simulink library "Lib_Piccolo"  (R2018b)
settings: Solver=VariableStepAuto  StartTime=0.0  StopTime=10.0  RelTol=1e-3
values from neighbouring files (symbols this model uses):
  AccelErrInt2Brakes = 0.15    [SimulationControlConfig16P.m]    (also in SimulationControlConfig16P_F0.m; SimulationControlConfig16P_F2.m; SimulationControlConfig16P_LEGACY.m; SimulationControlConfigTAILLESS.m = 0.2)
  AileronMax = 25    [SimulationControlConfig16P.m]    (also in SimulationControlConfig16P_F0.m; SimulationControlConfig16P_F2.m; SimulationControlConfig16P_LEGACY.m; SimulationControlConfigTAILLESS.m)
  AileronPower = 0.00268    [SimulationControlConfig16P.m]    (also in SimulationControlConfig16P_F0.m; SimulationControlConfig16P_F2.m; SimulationControlConfig16P_LEGACY.m; SimulationControlConfigTAILLESS.m = 0.002266)
  AileronSurfaceMax = 45    [SimulationControlConfig16P.m]    (also in SimulationControlConfig16P_F0.m; SimulationControlConfig16P_F2.m; SimulationControlConfig16P_LEGACY.m; SimulationControlConfigTAILLESS_CGAFT_F0.m = 25)
  AileronTrim = 0    [SimulationControlConfig16P.m]    (also in SimulationControlConfig16P_F0.m; SimulationControlConfig16P_F2.m; SimulationControlConfig16P_LEGACY.m; SimulationControlConfigTAILLESS.m)
  Alt = 1000 + TerrainHeight    [SimulationStateConfig.m]
  AltCruise_m = Alt * 0.3048    [SimulationControlConfig16P.m]    (also in SimulationControlConfig16P_F2.m; SimulationControlConfigTAILLESS.m = Alt/3.28084; SimulationControlConfigTAILLESS_CGAFT_F0.m = 640; SimulationControlConfigTAILLESS_CGFWD_F0.m = 640)
  AltitudeRate2PitchCmdIntegratorInit = 0.1    [SimulationControlPre.m]
  AltMax = 10000    [SimulationControlConfig16P.m]    (also in SimulationControlConfig16P_F0.m; SimulationControlConfig16P_F2.m; SimulationControlConfig16P_LEGACY.m; SimulationControlConfigTAILLESS.m)
  AltMaxAccel = 2.5    [SimulationControlConfig16P.m]    (also in SimulationControlConfig16P_F0.m = 2; SimulationControlConfig16P_F2.m = 2; SimulationControlConfig16P_LEGACY.m = 0.9; SimulationControlConfigTAILLESS.m = 2)
  AltMin = 0    [SimulationControlConfig16P.m]    (also in SimulationControlConfig16P_F0.m; SimulationControlConfig16P_F2.m; SimulationControlConfig16P_LEGACY.m; SimulationControlConfigTAILLESS.m)
  AltRateCmd2Pitch = 0.26    [SimulationControlConfig16P.m]    (also in SimulationControlConfig16P_F0.m = 0.35; SimulationControlConfig16P_F2.m = 0.35; SimulationControlConfig16P_LEGACY.m = 0.6; SimulationControlConfigTAILLESS.m = 0.9)
  AltRateError2Pitch = 0.34    [SimulationControlConfig16P.m]    (also in SimulationControlConfig16P_F0.m = 0.61; SimulationControlConfig16P_F2.m = 0.61; SimulationControlConfig16P_LEGACY.m = 0.4; SimulationControlConfigTAILLESS.m = 0.3)
  AltRateErrorInt2Pitch = 0.61    [SimulationControlConfig16P.m]    (also in SimulationControlConfig16P_F0.m = 0.28; SimulationControlConfig16P_F2.m = 0.28; SimulationControlConfig16P_LEGACY.m = 0.45; SimulationControlConfigTAILLESS.m = 0.15)
  AltRateLpfCutOff = 3    [SimulationControlConfig16P.m]    (also in SimulationControlConfig16P_F0.m; SimulationControlConfig16P_F2.m; SimulationControlConfig16P_LEGACY.m; SimulationControlConfigTAILLESS.m = 5)
  AutoNosegear2Rudder = 26    [SimulationControlConfig16P.m]    (also in SimulationControlConfig16P_F0.m; SimulationControlConfig16P_F2.m; SimulationControlConfig16P_LEGACY.m; SimulationControlConfigTAILLESS.m = 25.2)
  b = 5.54    [SimulationControlConfig16P.m]    (also in SimulationControlConfig16P_F0.m; SimulationControlConfig16P_F2.m; SimulationControlConfig16P_LEGACY.m; SimulationControlConfigTAILLESS.m = 2.37)
  Bank2AileronIntegratorInit = 0    [SimulationControlPre.m]
  BankMax_User = BankMax_User/180*pi    (= 0.610865238198)    [SimulationControlConfig16P.m]    (also in SimulationControlConfig16P_F0.m = 0.523598775598; SimulationControlConfig16P_F2.m = 0.523598775598; SimulationControlConfig16P_LEGACY.m = 0.523598775598; SimulationControlConfigTAILLESS.m = 0.558505360638)
  baseLegFlaps = 20    [SimulationControlConfig16P.m]    (also in SimulationControlConfig16P_F0.m; SimulationControlConfig16P_F2.m = 15; SimulationControlConfig16P_LEGACY.m = 0; SimulationControlConfigTAILLESS.m = 0)
  C = GeneticOpt.C    [SimulationCostFunction.m]
  c = Sw/b    (= 0.841696750903)    [SimulationControlConfig16P.m]    (also in SimulationControlConfig16P_F0.m; SimulationControlConfig16P_F2.m; SimulationControlConfig16P_LEGACY.m; SimulationControlConfigTAILLESS.m = 0.354008438819)
  cell2WheelFactorMG = 5.98    [SimulationSensorConfig16P_LEGACY.m]
  cell2WheelFactorNG = 1    [SimulationSensorConfig16P_LEGACY.m]
  cellSatMaxMG = 15000    [SimulationSensorConfig16P.m]    (also in SimulationSensorConfig16P_LEGACY.m; SimulationSensorConfigTAILLESS7P.m; SimulationSensorConfigUTAIL7P.m)
  cellSatMaxNG = 1000    [SimulationSensorConfig16P.m]    (also in SimulationSensorConfig16P_LEGACY.m; SimulationSensorConfigTAILLESS7P.m; SimulationSensorConfigUTAIL7P.m)
  cellSatMinMG = -15000    [SimulationSensorConfig16P.m]    (also in SimulationSensorConfig16P_LEGACY.m; SimulationSensorConfigTAILLESS7P.m; SimulationSensorConfigUTAIL7P.m)
  cellSatMinNG = -1000    [SimulationSensorConfig16P.m]    (also in SimulationSensorConfig16P_LEGACY.m; SimulationSensorConfigTAILLESS7P.m; SimulationSensorConfigUTAIL7P.m)
  CL_Limit = CL_Max    (= 0.54)    [SimulationControlConfig16P.m]    (also in SimulationControlConfig16P_F0.m; SimulationControlConfig16P_F2.m = 0.638; SimulationControlConfig16P_LEGACY.m; SimulationControlConfigTAILLESS.m = 0.525)
  CL_Max = 0.54    [SimulationControlConfig16P.m]    (also in SimulationControlConfig16P_F0.m; SimulationControlConfig16P_F2.m = 0.638; SimulationControlConfig16P_LEGACY.m; SimulationControlConfigTAILLESS.m = 0.525)
  CL_Max_Nom = 0.465    [SimulationControlConfig16P.m]    (also in SimulationControlConfig16P_F0.m; SimulationControlConfig16P_F2.m = 0.563; SimulationControlConfig16P_LEGACY.m; SimulationControlConfigTAILLESS.m = 0.39)
  CL_Min = 0    [SimulationControlConfig16P.m]    (also in SimulationControlConfig16P_F0.m; SimulationControlConfig16P_F2.m; SimulationControlConfig16P_LEGACY.m; SimulationControlConfigTAILLESS.m)
  ClimbMaxFraction = 0.35    [SimulationControlConfig16P.m]    (also in SimulationControlConfig16P_F0.m = 0.17; SimulationControlConfig16P_F2.m = 0.17; SimulationControlConfig16P_LEGACY.m = 0.24; SimulationControlConfigTAILLESS.m = 0.21)
  ClimboutMaxBank = 7.0    (= 7)    [SimulationControlConfig16P.m]    (also in SimulationControlConfig16P_F0.m; SimulationControlConfig16P_F2.m; SimulationControlConfig16P_LEGACY.m; SimulationControlConfigTAILLESS.m = 5)
  ClimboutTimer = 7.0    (= 7)    [SimulationControlConfig16P.m]    (also in SimulationControlConfig16P_F0.m; SimulationControlConfig16P_F2.m; SimulationControlConfig16P_LEGACY.m; SimulationControlConfigTAILLESS.m)
  dCl_per_dFlap = 0.005581818    [SimulationControlConfig16P.m]    (also in SimulationControlConfig16P_F0.m = 0; SimulationControlConfig16P_F2.m = 0.0065; SimulationControlConfig16P_LEGACY.m = 0; SimulationControlConfigTAILLESS.m = 0)
  DecelerationCmd = 3.1    [SimulationControlConfig16P.m]    (also in SimulationControlConfig16P_F0.m; SimulationControlConfig16P_F2.m; SimulationControlConfig16P_LEGACY.m; SimulationControlConfigTAILLESS.m = 0.1)
  DeRotateLogicEndTimer = abs((NoseDownLimit_Deg-1)/DeRotateRamp_Dps)    [SimulationControlConfig16P.m]    (also in SimulationControlConfig16P_F0.m; SimulationControlConfig16P_F2.m; SimulationControlConfig16P_LEGACY.m; SimulationControlConfigTAILLESS.m)
  DeRotateLogicHoldNoseUpTimer = 0.1    [SimulationControlConfig16P.m]    (also in SimulationControlConfig16P_F0.m; SimulationControlConfig16P_F2.m; SimulationControlConfig16P_LEGACY.m; SimulationControlConfigTAILLESS.m)
  DeRotateLogicTimerTimeout = 2    [SimulationControlConfig16P.m]    (also in SimulationControlConfig16P_F0.m; SimulationControlConfig16P_F2.m; SimulationControlConfig16P_LEGACY.m; SimulationControlConfigTAILLESS.m)
  DeRotateLowerCmdSaturation = 0    [SimulationControlConfig16P.m]    (also in SimulationControlConfig16P_F0.m; SimulationControlConfig16P_F2.m; SimulationControlConfig16P_LEGACY.m; SimulationControlConfigTAILLESS.m)
  DeRotateRamp_Dps = 3    [SimulationControlConfig16P.m]    (also in SimulationControlConfig16P_F0.m; SimulationControlConfig16P_F2.m; SimulationControlConfig16P_LEGACY.m; SimulationControlConfigTAILLESS.m = 8)
  DeRotateUpperCmdSaturation = 7    [SimulationControlConfig16P.m]    (also in SimulationControlConfig16P_F0.m; SimulationControlConfig16P_F2.m; SimulationControlConfig16P_LEGACY.m; SimulationControlConfigTAILLESS.m)
  DescentMaxFraction = 0.22    [SimulationControlConfig16P.m]    (also in SimulationControlConfig16P_F0.m = 0.2; SimulationControlConfig16P_F2.m = 0.2; SimulationControlConfig16P_LEGACY.m = 0.2; SimulationControlConfigTAILLESS.m = 0.17)
  DesktopSimTerrainOffset_m = 0.406    [SimulationAircraftConfig.m]
  downwindFlaps = 0    [SimulationControlConfig16P.m]    (also in SimulationControlConfig16P_F0.m; SimulationControlConfig16P_F2.m = 15; SimulationControlConfig16P_LEGACY.m; SimulationControlConfigTAILLESS.m)
  downwindSplitAil = 0    [SimulationControlConfig16P_F2.m]
  DP_init = 0.5*1.225*V_init^2    [SimulationControlConfig16P.m]    (also in SimulationControlConfig16P_F0.m; SimulationControlConfig16P_F2.m; SimulationControlConfig16P_LEGACY.m; SimulationControlConfigTAILLESS.m)
  dscNoiseMG = 1    [SimulationSensorConfig16P_LEGACY.m]
  dscNoiseNG = 0.25    [SimulationSensorConfig16P_LEGACY.m]
  DSCnumBits = 24    [SimulationSensorConfig16P.m]    (also in SimulationSensorConfig16P_LEGACY.m; SimulationSensorConfigTAILLESS7P.m; SimulationSensorConfigUTAIL7P.m)
  DSCRangeMaxMG = 15000    [SimulationSensorConfig16P.m]    (also in SimulationSensorConfig16P_LEGACY.m; SimulationSensorConfigTAILLESS7P.m; SimulationSensorConfigUTAIL7P.m)
  DSCRangeMaxNG = 1000    [SimulationSensorConfig16P.m]    (also in SimulationSensorConfig16P_LEGACY.m; SimulationSensorConfigTAILLESS7P.m; SimulationSensorConfigUTAIL7P.m)
  DSCRangeMinMG = -15000    [SimulationSensorConfig16P.m]    (also in SimulationSensorConfig16P_LEGACY.m; SimulationSensorConfigTAILLESS7P.m; SimulationSensorConfigUTAIL7P.m)
  DSCRangeMinNG = -1000    [SimulationSensorConfig16P.m]    (also in SimulationSensorConfig16P_LEGACY.m; SimulationSensorConfigTAILLESS7P.m; SimulationSensorConfigUTAIL7P.m)
  dt = DLLSim.dt    [SimulationTimeStep.m]    (also in SimulationTrim.m = 0.02)
  EarlyTouchdownThreshold = 3.0    (= 3)    [SimulationControlConfig16P.m]    (also in SimulationControlConfig16P_F0.m; SimulationControlConfig16P_F2.m; SimulationControlConfig16P_LEGACY.m; SimulationControlConfigTAILLESS.m)
  ElevatorDeflectionRate = 15    [SimulationControlConfig16P.m]    (also in SimulationControlConfig16P_F0.m; SimulationControlConfig16P_F2.m; SimulationControlConfig16P_LEGACY.m = 12; SimulationControlConfigTAILLESS.m = 5)
  ElevatorMax = 25    [SimulationControlConfig16P.m]    (also in SimulationControlConfig16P_F0.m; SimulationControlConfig16P_F2.m; SimulationControlConfig16P_LEGACY.m; SimulationControlConfigTAILLESS.m)
  ElevatorPower = -0.002209    [SimulationControlConfig16P.m]    (also in SimulationControlConfig16P_F0.m; SimulationControlConfig16P_F2.m; SimulationControlConfig16P_LEGACY.m; SimulationControlConfigTAILLESS.m = -0.002668)
  ElevatorTrim = -3.5    [SimulationControlConfig16P.m]    (also in SimulationControlConfig16P_F0.m; SimulationControlConfig16P_F2.m; SimulationControlConfig16P_LEGACY.m; SimulationControlConfigTAILLESS.m = -3)
  elevonBias = 0    [SimulationControlConfig16P.m]    (also in SimulationControlConfig16P_F0.m; SimulationControlConfig16P_F2.m; SimulationControlConfig16P_LEGACY.m; SimulationControlConfigTAILLESS.m)
  Enable_TAS_Protection = 0    [SimulationControlConfig16P.m]    (also in SimulationControlConfig16P_F0.m; SimulationControlConfig16P_F2.m; SimulationControlConfig16P_LEGACY.m; SimulationControlConfigTAILLESS.m)
  EnableCrossTrackAbort = 1    [SimulationControlConfig16P.m]    (also in SimulationControlConfigTAILLESS.m; SimulationControlConfigTAILLESS_CGAFT_F0.m; SimulationControlConfigTAILLESS_CGFWD_F0.m; SimulationControlConfigTAILLESS_CGFWD_F2.m)
  EnergyBandwidth = 0.04    [SimulationControlConfig16P.m]    (also in SimulationControlConfig16P_F0.m = 0.03; SimulationControlConfig16P_F2.m = 0.03; SimulationControlConfig16P_LEGACY.m = 0.02; SimulationControlConfigTAILLESS.m = 0.06)
  EngineLhFuelCut = 0    [SimulationAircraftConfig.m]
  EngineRhFuelCut = 0    [SimulationAircraftConfig.m]
  FastThrottleRate = 0.075    [SimulationControlConfig16P.m]    (also in SimulationControlConfig16P_F0.m = 0.05; SimulationControlConfig16P_F2.m = 0.05; SimulationControlConfig16P_LEGACY.m = 0.05; SimulationControlConfigTAILLESS.m = 0.1)
  FilterWarmUpTime = 2    [SimulationSensorConfig16P.m]    (also in SimulationSensorConfig16P_LEGACY.m; SimulationSensorConfigTAILLESS7P.m; SimulationSensorConfigUTAIL7P.m)
  finalApproachFlaps = 20    [SimulationControlConfig16P.m]    (also in SimulationControlConfig16P_F0.m; SimulationControlConfig16P_F2.m = 15; SimulationControlConfig16P_LEGACY.m = 0; SimulationControlConfigTAILLESS.m = 0)
  finalApproachSplitAil = 20    [SimulationControlConfig16P_F2.m]
  FinalDescentSlope_Deg = testPlans(testIndx).descentSlope    [SimulationControlConfig16P.m]    (also in SimulationControlConfig16P_F0.m; SimulationControlConfig16P_F2.m; SimulationControlConfig16P_LEGACY.m; SimulationControlConfigTAILLESS.m)
  flapMax = 0    [SimulationControlConfig16P.m]    (also in SimulationControlConfig16P_F0.m = 35; SimulationControlConfig16P_F2.m = 33; SimulationControlConfig16P_LEGACY.m; SimulationControlConfigTAILLESS.m)
  flapRate = 7.5    [SimulationControlConfig16P.m]    (also in SimulationControlConfig16P_F0.m; SimulationControlConfig16P_F2.m; SimulationControlConfig16P_LEGACY.m; SimulationControlConfigTAILLESS.m = 6.6)
  FlareHeight = 5    [SimulationControlConfig16P.m]    (also in SimulationControlConfig16P_F0.m; SimulationControlConfig16P_F2.m; SimulationControlConfig16P_LEGACY.m = 4.8; SimulationControlConfigTAILLESS.m = 2.75)
  FlareVerticalRate_mps = -0.4    [SimulationControlConfig16P.m]    (also in SimulationControlConfig16P_F0.m; SimulationControlConfig16P_F2.m; SimulationControlConfig16P_LEGACY.m = -0.5; SimulationControlConfigTAILLESS.m = -0.15)
  Fp_Aileron = 0.55*2*pi*RollRateLpfCutoff*dt    [SimulationControlConfig16P.m]    (also in SimulationControlConfig16P_F0.m; SimulationControlConfig16P_F2.m; SimulationControlConfig16P_LEGACY.m; SimulationControlConfigTAILLESS.m)
  Fp_Alt = 2*pi*0.55*AltBandwidth    (= 0.622035345411)    [SimulationControlConfig16P.m]    (also in SimulationControlConfig16P_F0.m; SimulationControlConfig16P_F2.m; SimulationControlConfig16P_LEGACY.m = 0.099; SimulationControlConfigTAILLESS.m = 0.207345115137)
  Fp_AltRate = 0.55*2*pi*AltRateLpfCutOff*dt    [SimulationControlConfig16P.m]    (also in SimulationControlConfig16P_F0.m; SimulationControlConfig16P_F2.m; SimulationControlConfig16P_LEGACY.m; SimulationControlConfigTAILLESS.m)
  Fp_Elevator = 0.55*2*pi*PitchRateLpfCutoff*dt    [SimulationControlConfig16P.m]    (also in SimulationControlConfig16P_F0.m; SimulationControlConfig16P_F2.m; SimulationControlConfig16P_LEGACY.m; SimulationControlConfigTAILLESS.m)
  Fp_Energy = 0.55*2*pi*EnergyBandwidth    (= 0.138230076758)    [SimulationControlConfig16P.m]    (also in SimulationControlConfig16P_F0.m = 0.103672557568; SimulationControlConfig16P_F2.m = 0.103672557568; SimulationControlConfig16P_LEGACY.m = 0.069115038379; SimulationControlConfigTAILLESS.m = 0.207345115137)
  Fp_Energy2 = 0.55*2*pi*EnergyBandwidth*dt    [SimulationControlConfig16P.m]    (also in SimulationControlConfig16P_F0.m; SimulationControlConfig16P_F2.m; SimulationControlConfig16P_LEGACY.m; SimulationControlConfigTAILLESS.m)
  Fp_Pitch = 0.55*2*pi*PitchBandwidth    (= 2.45358386245)    [SimulationControlConfig16P.m]    (also in SimulationControlConfig16P_F0.m; SimulationControlConfig16P_F2.m = 1.72787595947; SimulationControlConfig16P_LEGACY.m = 3.11017672705; SimulationControlConfigTAILLESS.m = 1.55508836353)
  Fp_Pitch_2 = 0.55*2*pi*PitchBandwidth*dt    [SimulationControlConfig16P.m]    (also in SimulationControlConfig16P_F0.m; SimulationControlConfig16P_F2.m; SimulationControlConfig16P_LEGACY.m; SimulationControlConfigTAILLESS.m)
  Fp_Roll = RollBandwidth^2    (= 1.69)    [SimulationControlConfig16P.m]    (also in SimulationControlConfig16P_F0.m = 1.44; SimulationControlConfig16P_F2.m = 1.44; SimulationControlConfig16P_LEGACY.m = 1.44; SimulationControlConfigTAILLESS.m = 1.21)
  Fp_Rudder = 0.55*2*pi*YawRateLpfCutoff*dt    [SimulationControlConfig16P.m]    (also in SimulationControlConfig16P_F0.m; SimulationControlConfig16P_F2.m; SimulationControlConfig16P_LEGACY.m; SimulationControlConfigTAILLESS.m)
  Fp_TAS = 0.55*2*pi*TASBandwidth    (= 0.103672557568)    [SimulationControlConfig16P.m]    (also in SimulationControlConfig16P_F0.m; SimulationControlConfig16P_F2.m; SimulationControlConfig16P_LEGACY.m; SimulationControlConfigTAILLESS.m = 0.172787595947)
  Fp_TAS_Filter = 2*pi*TasLpfCutoff*dt    [SimulationControlConfig16P.m]    (also in SimulationControlConfig16P_F0.m; SimulationControlConfig16P_F2.m; SimulationControlConfig16P_LEGACY.m; SimulationControlConfigTAILLESS.m)
  Fp_Turn = 0.55*2*pi*TurnErrLPFcutoff    (= 0.172787595947)    [SimulationControlConfig16P.m]    (also in SimulationControlConfig16P_F0.m = 0.0345575191895; SimulationControlConfig16P_F2.m = 0.0345575191895; SimulationControlConfig16P_LEGACY.m = 0.0345575191895; SimulationControlConfigTAILLESS.m)
  Fp_TurnDerr = 0.55*2*pi*TurnDerivativeLPFcutoff    (= 0.172787595947)    [SimulationControlConfig16P.m]    (also in SimulationControlConfig16P_F0.m = 0.0345575191895; SimulationControlConfig16P_F2.m = 0.0345575191895; SimulationControlConfig16P_LEGACY.m = 0.0345575191895; SimulationControlConfigTAILLESS.m)
  FTV = 3    [SimulationAircraftConfig.m]
  ftvStaticPositionError = 1/1.18    (= 0.847457627119)    [SimulationSensorConfig16P.m]    (also in SimulationSensorConfig16P_LEGACY.m; SimulationSensorConfigTAILLESS7P.m = 1; SimulationSensorConfigUTAIL7P.m = 1)
  g = 9.81    [SimulationStateConfig.m]
  goAroundSplitAil = 0    [SimulationControlConfig16P_F2.m]
  GustSpd_Kts = testPlans(testIndx).gustSpd    [SimulationStateConfig.m]
  GustTriggerVal = testPlans(testIndx).gustTriggerVal    [SimulationStateConfig.m]
  HeadingErr2TurnRate = 0.5    [SimulationControlConfig16P.m]    (also in SimulationControlConfig16P_F0.m; SimulationControlConfig16P_F2.m; SimulationControlConfig16P_LEGACY.m; SimulationControlConfigTAILLESS.m)
  HeadingErrDer2TurnRate = 0.3    [SimulationControlConfig16P.m]    (also in SimulationControlConfig16P_F0.m; SimulationControlConfig16P_F2.m; SimulationControlConfig16P_LEGACY.m; SimulationControlConfigTAILLESS.m)
  IASbounce = IASstall*0.8    [SimulationControlPre.m]
  IAScruiseCMD = sqrt(2*m*9.81/(1.225*Sw*CL_cruise))    [SimulationControlConfig16P.m]    (also in SimulationControlConfig16P_F0.m; SimulationControlConfig16P_F2.m; SimulationControlConfig16P_LEGACY.m; SimulationControlConfigTAILLESS.m)
  IASfinalCMD = 1.12 * IASmin    [SimulationControlConfig16P.m]    (also in SimulationControlConfig16P_F0.m = 1.14 * IASmin; SimulationControlConfig16P_F2.m = 1.10 * IASmin; SimulationControlConfig16P_LEGACY.m = 1.10 * IASmin; SimulationControlConfigTAILLESS.m = 1.14 * IASmin)
  IASflareCMD = IASstall    [SimulationControlConfig16P.m]    (also in SimulationControlConfig16P_F0.m; SimulationControlConfig16P_F2.m; SimulationControlConfig16P_LEGACY.m; SimulationControlConfigTAILLESS.m)
  IASmax = 64    [SimulationControlConfig16P.m]    (also in SimulationControlConfig16P_F0.m = 46; SimulationControlConfig16P_F2.m = 52; SimulationControlConfig16P_LEGACY.m = 46; SimulationControlConfigTAILLESS.m = 38.9)
  IASmin = sqrt(2*m*9.81/(1.225*Sw*0.9*CL_Max_Nom))    [SimulationControlConfig16P.m]    (also in SimulationControlConfig16P_F0.m; SimulationControlConfig16P_F2.m; SimulationControlConfig16P_LEGACY.m; SimulationControlConfigTAILLESS.m)
  IASshortCMD = IASstall    [SimulationControlConfig16P.m]    (also in SimulationControlConfig16P_F0.m; SimulationControlConfig16P_F2.m; SimulationControlConfig16P_LEGACY.m; SimulationControlConfigTAILLESS.m)
  IASstall = sqrt(2*m*9.81/(1.225*Sw*CL_Max))    [SimulationControlConfig16P.m]    (also in SimulationControlConfig16P_F0.m; SimulationControlConfig16P_F2.m; SimulationControlConfig16P_LEGACY.m; SimulationControlConfigTAILLESS.m)
  inFlight = 1    [SimulationControlConfig16P.m]    (also in SimulationControlConfigTAILLESS.m; SimulationControlConfigTAILLESS_CGAFT_F0.m; SimulationControlConfigTAILLESS_CGFWD_F0.m; SimulationControlConfigTAILLESS_CGFWD_F2.m)
  JetCatOffset = 5    [SimulationControlConfig16P.m]    (also in SimulationControlConfig16P_F0.m; SimulationControlConfig16P_F2.m; SimulationControlConfig16P_LEGACY.m)
  LaunchRollingElevator = -1.5    [SimulationControlConfig16P.m]    (also in SimulationControlConfig16P_F0.m; SimulationControlConfig16P_F2.m = 1.25; SimulationControlConfig16P_LEGACY.m; SimulationControlConfigTAILLESS.m = 1)
  ldg_NosegearMax = 10    [SimulationControlConfig16P.m]    (also in SimulationControlConfig16P_F0.m; SimulationControlConfig16P_F2.m; SimulationControlConfig16P_LEGACY.m; SimulationControlConfigTAILLESS.m)
  ldg_TrackVyErrInt2Nosegear = 0.1250    (= 0.125)    [SimulationControlConfig16P.m]    (also in SimulationControlConfig16P_F0.m; SimulationControlConfig16P_F2.m; SimulationControlConfig16P_LEGACY.m; SimulationControlConfigTAILLESS.m = 0.00714285714286)
  ldg_TrackVyErrPro2Nosegear = 0.35    [SimulationControlConfig16P.m]    (also in SimulationControlConfig16P_F0.m; SimulationControlConfig16P_F2.m; SimulationControlConfig16P_LEGACY.m; SimulationControlConfigTAILLESS.m = 0.0546666666667)
  ldg_TrackY2Vy = 0.07    [SimulationControlConfig16P.m]    (also in SimulationControlConfig16P_F0.m; SimulationControlConfig16P_F2.m; SimulationControlConfig16P_LEGACY.m; SimulationControlConfigTAILLESS.m = 0.17)
  ldg_Vy2NosegearScalingPower = 1.075    [SimulationControlConfig16P.m]    (also in SimulationControlConfig16P_F0.m; SimulationControlConfig16P_F2.m; SimulationControlConfig16P_LEGACY.m; SimulationControlConfigTAILLESS.m = 0.6)
  ldg_Y2VyScalingPower = 0.175    [SimulationControlConfig16P.m]    (also in SimulationControlConfig16P_F0.m; SimulationControlConfig16P_F2.m; SimulationControlConfig16P_LEGACY.m; SimulationControlConfigTAILLESS.m = 0)
  ldg_YawRate2Nosegear = 0.175    [SimulationControlConfig16P.m]    (also in SimulationControlConfig16P_F0.m; SimulationControlConfig16P_F2.m; SimulationControlConfig16P_LEGACY.m; SimulationControlConfigTAILLESS.m = 0.065)
  LiftSlope = 0.064285    [SimulationControlConfig16P.m]    (also in SimulationControlConfig16P_F0.m; SimulationControlConfig16P_F2.m; SimulationControlConfig16P_LEGACY.m; SimulationControlConfigTAILLESS.m = 0.058631)
  LPFaileronInit = 0    [SimulationControlPre.m]
  LPFclestInit = 0    [SimulationControlPre.m]
  LPFenergyFFInit = 0    [SimulationControlPre.m]
  ... (+122 more)
undefined symbols (not defined in the file or in its folder): abortFlag, alphaHPF, apmDelay, BRWNOUT, CRAWOR, CRAWUR, DiscIntNeverNeededParam, DLLSim, DLLSimStep, ECOMOR, ECOMUR, Fp_Tas, GustTrigger_HeightAgl_m, IPSTAT, LCINTEG, Ldg_Persist_Time, LOWER_FLAGS, MSG_ENABLE, NoiseStd, OLDVAL, OVERRIDE_ENABLE, OVERRIDE_VALUE, REBOOT, reversionEnable, revIASMax, revIASMin, revPitchMax, revPitchMin, revPitchRateMax, revRollMax, revRollRateMax, SAMPLE, SCALON, SensorModel, sigbuilder_block, Sim_Vx, Sim_Vy, Sim_Vz, Sim_Xpos, Sim_Ypos, Sim_Zpos, SYSOR, SYSUR, TARE, TEMPOR, TEMPUR, testIndx, testPlan, testPlans, Trim_piccoloInCmd, Trim_REFSI_FD_IN_nmodeCgShifterCmd_Flag, Trim_REFSI_FD_IN_nmodeCgShifterCmd_Ft, Trim_REFSI_FD_IN_nmodeCgShifterCmdType, Trim_REFSI_FD_IN_nmodeCgShifterNRCActive, Trim_REFSI_FD_IN_nmodeFlapLhIBCmd_Deg, Trim_REFSI_FD_IN_nmodeFlapLhOBCmd_Deg, Trim_REFSI_FD_IN_nmodeFlapRhIBCmd_Deg, Trim_REFSI_FD_IN_nmodeFlapRhOBCmd_Deg, Trim_REFSI_FD_IN_nmodeSlatLhCmd_Deg ... (+11)
libraries: simulink x1237, $bdroot x179, aerolibconvert2 x63, dspswit3 x25, aerolibatmos2 x5, simulink_extras x4, dsparch4 x2, Lib_Piccolo_Alt x2, eeGeneralControl x1, dspindex x1
(part 24 of 74)

== system Lib_Piccolo/Emulated INS/Accelerometer Noise Model/Generate Accel Noise ==
  ContactBool : Inport
  gndSpeed_mps : Inport  Port=2
  Constant1 : Constant
  Constant2 : Constant  Value=10
  Data Type Conversion : DataTypeConversion
  Divide : Product  Inputs=*/
  Low-Pass Filter (Discrete or Continuous) : eeGeneralControl/Low-Pass Filter (Discrete or Continuous)  Commented=through  K=1  T=0.2  B=inf  A=-inf  init_option=Inherited from block input  x0=0  Ts=-1
  Multiply{,1..8} (9 alike) : Product
  Saturation3 : Saturate  UpperLimit=SensorModel.IMU.noiseScalarMax  LowerLimit=SensorModel.IMU.noiseScalarMin
  Sum : Sum  Inputs=+-|
  Sum1 : Sum
  Sum2 : Sum
  Sum3 : Sum
  xAccelNoiseInAir : RandomNumber  Variance=SensorModel.IMU.xAccelNoiseVarianceInAir
  xAccelNoiseOnGnd : RandomNumber  Variance=SensorModel.IMU.xAccelNoiseVarianceOnGnd
  yAccelNoiseInAir : RandomNumber  Variance=SensorModel.IMU.yAccelNoiseVarianceInAir
  yAccelNoiseOnGnd : RandomNumber  Variance=SensorModel.IMU.yAccelNoiseVarianceOnGnd
  zAccelNoiseInAir : RandomNumber  Variance=SensorModel.IMU.zAccelNoiseVarianceInAir
  zAccelNoiseOnGnd : RandomNumber  Variance=SensorModel.IMU.zAccelNoiseVarianceOnGnd
  NoiseXaccelmps2 : Outport
  NoiseYaccelmps2 : Outport  Port=2
  NoiseZaccelmps2 : Outport  Port=3
  wires:
  Sum1/1 -> Multiply8/1
  Multiply8/1 -> NoiseXaccelmps2/1
  Multiply7/1 -> NoiseYaccelmps2/1
  Sum2/1 -> Multiply7/1
  Multiply6/1 -> NoiseZaccelmps2/1
  Sum3/1 -> Multiply6/1
  Saturation3/1 -> Multiply6/2, Multiply7/2, Multiply8/2  "gndSpdScalar"
  Constant2/1 -> Divide/2
  Divide/1 -> Saturation3/1
  gndSpeed_mps/1 -> Divide/1
  ContactBool/1 -> Data Type Conversion/1
  Data Type Conversion/1 -> Low-Pass Filter (Discrete or Continuous)/1
  zAccelNoiseInAir/1 -> Multiply4/1
  Multiply5/1 -> Sum3/2
  Multiply4/1 -> Sum3/1
  zAccelNoiseOnGnd/1 -> Multiply5/2
  Multiply2/1 -> Sum2/1
  yAccelNoiseOnGnd/1 -> Multiply3/2
  yAccelNoiseInAir/1 -> Multiply2/1
  Multiply3/1 -> Sum2/2
  xAccelNoiseOnGnd/1 -> Multiply1/2
  xAccelNoiseInAir/1 -> Multiply/1
  Multiply1/1 -> Sum1/2
  Constant1/1 -> Sum/1
  Low-Pass Filter (Discrete or Continuous)/1 -> Sum/2, Multiply1/1, Multiply3/1, Multiply5/1  "onGnd"
  Sum/1 -> Multiply2/2, Multiply4/2, Multiply/2  "inAir"
  Multiply/1 -> Sum1/1

== system Lib_Piccolo/Ground Detection Systems/CL Detection Wrapper/CL Based Touchdown Detection Logic ==
  note: This is a latch used only in the touchdown, and rollout Piccolo Controller Modes
  note: When this is true Piccolo is indicating the WOW system armed.
  note: This is a latch used only in the short final, touchdown, and rollout Piccolo Controller Modes
  Pic_WOW : Inport
  Pic_APMode : Inport  Port=2
  CL : Inport  Port=3
  Compare To Constant1 : simulink/Logic and Bit Operations/Compare To Constant  relop=>  const=-1  OutDataTypeStr=uint8
  Compare To Constant2 : simulink/Logic and Bit Operations/Compare To Constant  relop=>=  const=10  OutDataTypeStr=uint8
  Compare To Constant6 : simulink/Logic and Bit Operations/Compare To Constant  relop=>=  const=9  OutDataTypeStr=uint8
  Constant : Constant  Value=EarlyTouchdownThreshold
  Constant1 : Constant  Value=TouchdownThreshold
  Constant10 : Constant  Value=0
  Constant2 : Constant  Value=CL_Max
  Constant3 : Constant  Value=0
  Constant4 : Constant
  Constant5 : Constant
  Constant6 : Constant  Value=0
  Constant7 : Constant  Value=TouchdownThreshold
  Constant8 : Constant  Value=2
  Constant9 : Constant
  Latch : Subsystem
  Latch1 : Subsystem
  Multiply{,1..4} (5 alike) : Product
  NOT : Logic  Operator=NOT  IconShape=distinctive  AllPortsSameDT=off  OutDataTypeStr=boolean
  Subtract : Sum  Inputs=-+
  Subtract1 : Sum  Inputs=-+
  Subtract2 : Sum  Inputs=+-
  Switch : Switch
  Switch1 : Switch
  Switch2 : Switch  Threshold=2
  Switch3 : Switch
  Switch4 : Switch  Criteria=u2 > Threshold
  EarlyTouchdownFlag : Outport
  TouchdownFlag : Outport  Port=2
  wires:
  Pic_WOW/1 -> Compare To Constant1/1
  Compare To Constant1/1 -> NOT/1
  Switch/1 -> Switch4/1
  Switch3/1 -> Switch4/3
  Constant5/1 -> Switch1/1
  Constant6/1 -> Switch1/3
  Constant4/1 -> Switch/1
  Multiply/1 -> Subtract1/1
  Constant1/1 -> Multiply1/2
  Constant/1 -> Multiply/2
  Constant3/1 -> Switch/3
  Subtract/1 -> Switch/2
  Subtract1/1 -> Switch1/2
  CL/1 -> Subtract2/1, Subtract1/2, Subtract/2
  Constant2/1 -> Multiply/1, Multiply2/1, Multiply1/1
  Multiply1/1 -> Subtract/1
  Constant7/1 -> Switch2/1, Switch2/2
  Switch2/1 -> Multiply2/2
  Multiply2/1 -> Subtract2/2
  Subtract2/1 -> Switch3/2
  Constant9/1 -> Switch3/1
  Constant10/1 -> Switch3/3
  Pic_APMode/1 -> Compare To Constant2/1, Compare To Constant6/1
  Switch1/1 -> Multiply3/1
  Constant8/1 -> Switch2/3
  NOT/1 -> Switch4/2
  Latch/1(Q_Latched) -> EarlyTouchdownFlag/1
  Latch1/1(Q_Latched) -> TouchdownFlag/1
  Compare To Constant2/1 -> Latch1/2(Enable/!Rst), Multiply4/2
  Compare To Constant6/1 -> Latch/2(Enable/!Rst), Multiply3/2
  Multiply3/1 -> Latch/1(D)
  Multiply4/1 -> Latch1/1(D)
  Switch4/1 -> Multiply4/1

== system Lib_Piccolo/Ground Detection Systems/WoW Wrapper/Variant Subsystem ==
  note: 16 - Logic derived from LOAD2, with key changes:
      | - Saturation on inputs to filter to prevent 'wind-up'
      | - Fix to signal probe location used to drive one-wheel and persistence chain (this is a change from LOAD14)
      |
      | NOTE - this variant of the model has updates & simplifications to model elements upstream of the K2 and correct representation of DSC resolution. Not propagated to previous variants!
  note: 1) Add Subsystem or Model blocks as valid variant choices.
      | 2) You cannot connect blocks at this level. At simulation, connectivity is automatically
      | determined, based on the active variant and port name matching.
  note: 18 - Core logic & modelling is matched to 16 , with updates to accomodate landing with single-wheel DSC failures.
  note: 20 - Detection logic is that of 16 with addition of single-wheel failure handling . System further developed in Simulink for test & code-generation capability.
  Piccolo_AP_Mode : Inport
  WoW_Bus_In : Inport  Port=2
  Load Cell WoW Model 1 : Subsystem  VariantControl="SensorModel.WOW.Cell.Variant==\"LOAD1\""  mask{Ldg_Persist_Time=SensorModel.WOW.Cell.persistanceTime_s, Ldg_Latch_Time_P=SensorModel.WOW.Cell.longLatchTime_s, Ldg_Latch_Time_S=SensorModel.WOW.Cell.shortLatchTime_s, Ldg_Load_Thresh_Upper=SensorModel.WOW.Cell.loadThresholdUpper_N, Ldg_Load_Thresh_Lower=SensorModel.WOW.Cell.loadThresholdLower_N, TO_Persist_Time=SensorModel.WOW.Cell.TO_persistanceTime_s, TO_Latch_Time=SensorModel.WOW.Cell.TO_latchTime_s, TO_Load_Thresh=SensorModel.WOW.Cell.TO_loadThreshold_N, DSCnumBits=24, numBits=16, satMaxMG=15000, satMinMG=-300, dscNoiseMG=1, DSCRangeMaxMG=15000, DSCRangeMinMG=-15000, satMaxNG=1000, satMinNG=-250, dscNoiseNG=0.25, DSCRangeMaxNG=1000, DSCRangeMinNG=-1000, cellSatMaxMG=15000, cellSatMinMG=-15000, cell2WheelFactorMG=5.98, cellSatMaxNG=1000, cellSatMinNG=-1000, cell2WheelFactorNG=1}
      mask prompts: Ldg_Persist_Time "Landing Persistance Time [s]"; Ldg_Latch_Time_P "Primary Landing Latch Time [s]"; Ldg_Latch_Time_S "Secondary Landing Latch Time [s]"; Ldg_Load_Thresh_Upper "Landing Load Threshold Upper [N]"; Ldg_Load_Thresh_Lower "Landing Load Threshold Lower [N]"; TO_Persist_Time "Take Off Persistance Time [s]"; TO_Latch_Time "Take Off Latch Time [s]"; TO_Load_Thresh "Take Off Load Threshold  [N]"; DSCnumBits "DSC Encoded Resolution [num bits]"; numBits "CANBridge Encoded Resolution [num bits]"; satMaxMG "Main Gear CANBridge Saturation Max [N]"; satMinMG "Main Gear CANBridge Saturation Min [N]"; dscNoiseMG "Main Gear DSC Noise Level pk-pk [N]"; DSCRangeMaxMG "Main Gear DSC Range Max [N]"; DSCRangeMinMG "Main Gear DSC Range Min [N]"; satMaxNG "Nose Gear CANBridge Saturation Max [N]"; satMinNG "Nose Gear CANBridge Saturation Min [N]"; dscNoiseNG "Nose Gear DSC Noise Level pk-pk [N]"; DSCRangeMaxNG "Nose Gear DSC Range Max [N]"; DSCRangeMinNG "Nose Gear DSC Range Min [N]"; cellSatMaxMG "Main Gear Cell Saturation Max [N]"; cellSatMinMG "Main Gear Cell Saturation Min [N]"; cell2WheelFactorMG "Main Gear Cell to Wheel Load Scale Factor"; cellSatMaxNG "Nose Gear Cell Saturation Max [N]"; cellSatMinNG "Nose Gear Cell Saturation Min [N]"; cell2WheelFactorNG "Nose Gear Cell to Wheel Load Scale Factor"
      mask DialogControl DescGroupVar Prompt: Full model of load-cell based weight-on-wheels system.
      mask DialogControl LogicGroupVar Prompt: Logic Configuration
      mask DialogControl DataGroupVar Prompt: Data Acquisition
      mask DialogControl Container5 Prompt: MG
      mask DialogControl Container6 Prompt: NG
      mask DialogControl ParamGroupVar Prompt: Physical Parameters
      mask DialogControl Container8 Prompt: MG
      mask DialogControl Container9 Prompt: NG
  Load Cell WoW Model 1 16P5 AsFlown 2022 : Subsystem  VariantControl="SensorModel.WOW.Cell.Variant==\"LOAD1_16P5_ASFLOWN\""  mask{Ldg_Persist_Time=0.06, Ldg_Latch_Time_P=0.7, Ldg_Latch_Time_S=0.4, Ldg_Load_Thresh_Upper=85, Ldg_Load_Thresh_Lower=27, TO_Persist_Time=0.02, TO_Latch_Time=0.5, TO_Load_Thresh=275, DSCnumBits=24, numBits=16, satMaxMG=15000, satMinMG=-300, dscNoiseMG=1, DSCRangeMaxMG=15000, DSCRangeMinMG=-15000, satMaxNG=1000, satMinNG=-250, dscNoiseNG=0.25, DSCRangeMaxNG=1000, DSCRangeMinNG=-1000, cellSatMaxMG=15000, cellSatMinMG=-15000, cell2WheelFactorMG=5.98, cellSatMaxNG=1000, cellSatMinNG=-1000, cell2WheelFactorNG=1}
      mask prompts: Ldg_Persist_Time "Landing Persistance Time [s]"; Ldg_Latch_Time_P "Primary Landing Latch Time [s]"; Ldg_Latch_Time_S "Secondary Landing Latch Time [s]"; Ldg_Load_Thresh_Upper "Landing Load Threshold Upper [N]"; Ldg_Load_Thresh_Lower "Landing Load Threshold Lower [N]"; TO_Persist_Time "Take Off Persistance Time [s]"; TO_Latch_Time "Take Off Latch Time [s]"; TO_Load_Thresh "Take Off Load Threshold  [N]"; DSCnumBits "DSC Encoded Resolution [num bits]"; numBits "CANBridge Encoded Resolution [num bits]"; satMaxMG "Main Gear CANBridge Saturation Max [N]"; satMinMG "Main Gear CANBridge Saturation Min [N]"; dscNoiseMG "Main Gear DSC Noise Level pk-pk [N]"; DSCRangeMaxMG "Main Gear DSC Range Max [N]"; DSCRangeMinMG "Main Gear DSC Range Min [N]"; satMaxNG "Nose Gear CANBridge Saturation Max [N]"; satMinNG "Nose Gear CANBridge Saturation Min [N]"; dscNoiseNG "Nose Gear DSC Noise Level pk-pk [N]"; DSCRangeMaxNG "Nose Gear DSC Range Max [N]"; DSCRangeMinNG "Nose Gear DSC Range Min [N]"; cellSatMaxMG "Main Gear Cell Saturation Max [N]"; cellSatMinMG "Main Gear Cell Saturation Min [N]"; cell2WheelFactorMG "Main Gear Cell to Wheel Load Scale Factor"; cellSatMaxNG "Nose Gear Cell Saturation Max [N]"; cellSatMinNG "Nose Gear Cell Saturation Min [N]"; cell2WheelFactorNG "Nose Gear Cell to Wheel Load Scale Factor"
      mask DialogControl DescGroupVar Prompt: Full model of load-cell based weight-on-wheels system.
      mask DialogControl LogicGroupVar Prompt: Logic Configuration
      mask DialogControl DataGroupVar Prompt: Data Acquisition
      mask DialogControl Container5 Prompt: MG
      mask DialogControl Container6 Prompt: NG
      mask DialogControl ParamGroupVar Prompt: Physical Parameters
      mask DialogControl Container8 Prompt: MG
      mask DialogControl Container9 Prompt: NG
  Load Cell WoW Model 1 7P AsFlown : Subsystem  VariantControl="SensorModel.WOW.Cell.Variant==\"LOAD1_7P_ASFLOWN\""  mask{Ldg_Persist_Time=0.06, Ldg_Latch_Time_P=0.5, Ldg_Latch_Time_S=0.5, Ldg_Load_Thresh_Upper=10, Ldg_Load_Thresh_Lower=3.5, TO_Persist_Time=0.02, TO_Latch_Time=0.5, TO_Load_Thresh=21.15, DSCnumBits=24, numBits=16, satMaxMG=15000, satMinMG=-300, dscNoiseMG=1, DSCRangeMaxMG=15000, DSCRangeMinMG=-15000, satMaxNG=1000, satMinNG=-250, dscNoiseNG=0.25, DSCRangeMaxNG=1000, DSCRangeMinNG=-1000, cellSatMaxMG=15000, cellSatMinMG=-15000, cell2WheelFactorMG=5.98, cellSatMaxNG=1000, cellSatMinNG=-1000, cell2WheelFactorNG=1}
      mask prompts: Ldg_Persist_Time "Landing Persistance Time [s]"; Ldg_Latch_Time_P "Primary Landing Latch Time [s]"; Ldg_Latch_Time_S "Secondary Landing Latch Time [s]"; Ldg_Load_Thresh_Upper "Landing Load Threshold Upper [N]"; Ldg_Load_Thresh_Lower "Landing Load Threshold Lower [N]"; TO_Persist_Time "Take Off Persistance Time [s]"; TO_Latch_Time "Take Off Latch Time [s]"; TO_Load_Thresh "Take Off Load Threshold  [N]"; DSCnumBits "DSC Encoded Resolution [num bits]"; numBits "CANBridge Encoded Resolution [num bits]"; satMaxMG "Main Gear CANBridge Saturation Max [N]"; satMinMG "Main Gear CANBridge Saturation Min [N]"; dscNoiseMG "Main Gear DSC Noise Level pk-pk [N]"; DSCRangeMaxMG "Main Gear DSC Range Max [N]"; DSCRangeMinMG "Main Gear DSC Range Min [N]"; satMaxNG "Nose Gear CANBridge Saturation Max [N]"; satMinNG "Nose Gear CANBridge Saturation Min [N]"; dscNoiseNG "Nose Gear DSC Noise Level pk-pk [N]"; DSCRangeMaxNG "Nose Gear DSC Range Max [N]"; DSCRangeMinNG "Nose Gear DSC Range Min [N]"; cellSatMaxMG "Main Gear Cell Saturation Max [N]"; cellSatMinMG "Main Gear Cell Saturation Min [N]"; cell2WheelFactorMG "Main Gear Cell to Wheel Load Scale Factor"; cellSatMaxNG "Nose Gear Cell Saturation Max [N]"; cellSatMinNG "Nose Gear Cell Saturation Min [N]"; cell2WheelFactorNG "Nose Gear Cell to Wheel Load Scale Factor"
      mask DialogControl DescGroupVar Prompt: Full model of load-cell based weight-on-wheels system.
      mask DialogControl LogicGroupVar Prompt: Logic Configuration
      mask DialogControl DataGroupVar Prompt: Data Acquisition
      mask DialogControl Container5 Prompt: MG
      mask DialogControl Container6 Prompt: NG
      mask DialogControl ParamGroupVar Prompt: Physical Parameters
      mask DialogControl Container8 Prompt: MG
      mask DialogControl Container9 Prompt: NG
  Load Cell WoW Model 15 : Subsystem  VariantControl="SensorModel.WOW.Cell.Variant==\"LOAD15\""
  Load Cell WoW Model 16 : Subsystem  VariantControl="SensorModel.WOW.Cell.Variant==\"LOAD16\""
  Load Cell WoW Model 18 : Subsystem  VariantControl="SensorModel.WOW.Cell.Variant==\"LOAD18\""
  Load Cell WoW Model 20 : Subsystem  VariantControl="SensorModel.WOW.Cell.Variant==\"LOAD20\""
  Load Cell WoW Model 21 : Subsystem  VariantControl="SensorModel.WOW.Cell.Variant==\"LOAD21\""
  Load Cell WoW Model 22 : Subsystem  VariantControl="SensorModel.WOW.Cell.Variant==\"LOAD22\""
  Load Cell WoW Model 23 : Subsystem  VariantControl="SensorModel.WOW.Cell.Variant==\"LOAD23\""
  Load Cell WoW Model 24 : Subsystem  VariantControl="SensorModel.WOW.Cell.Variant==\"LOAD24\""
  WOW_Bus_Out : Outport

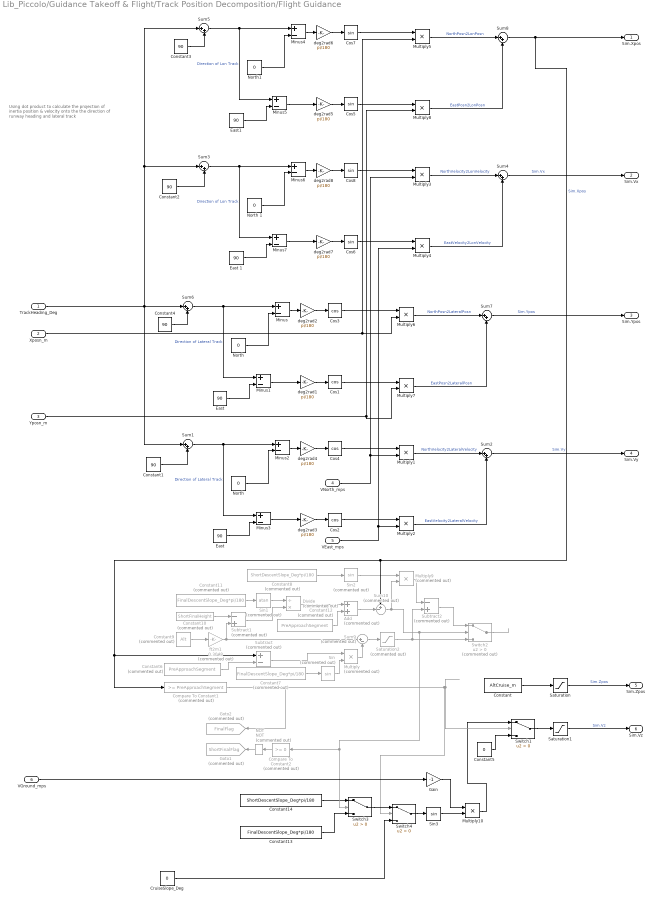
== system Lib_Piccolo/Guidance Takeoff & Flight/Track Position Decomposition/Flight Guidance ==
  note: Using dot product to calculate the projection of inertia position & velocity onto the
      | the direction of runway heading and lateral track
  TrackHeading_Deg : Inport
  Xposn_m : Inport  Port=2
  Yposn_m : Inport  Port=3
  VNorth_mps : Inport  Port=4
  VEast_mps : Inport  Port=5
  VGround_mps : Inport  Port=6
  Add : Sum  Commented=on
  Compare To Constant1 : simulink/Logic and Bit Operations/Compare To Constant  Commented=on  relop=>=  const=PreApproachSegment  OutDataTypeStr=uint8
  Compare To Constant2 : simulink/Logic and Bit Operations/Compare To Constant  Commented=on  relop=>=  const=0  OutDataTypeStr=uint8
  Constant : Constant  Value=AltCruise_m
  Constant{1..4} (4 alike) : Constant  Value=90
  Constant10 : Constant  Commented=on  Value=ShortFinalHeight
  Constant11 : Constant  Commented=on  Value=FinalDescentSlope_Deg*pi/180
  Constant12 : Constant  Commented=on  Value=PreApproachSegment
  Constant13 : Constant  Value=FinalDescentSlope_Deg*pi/180
  Constant14 : Constant  Value=ShortDescentSlope_Deg*pi/180
  Constant5 : Constant  Value=0
  Constant6 : Constant  Commented=on  Value=PreApproachSegment
  Constant7 : Constant  Commented=on  Value=FinalDescentSlope_Deg*pi/180
  Constant8 : Constant  Commented=on  Value=ShortDescentSlope_Deg*pi/180
  Constant9 : Constant  Commented=on  Value=Alt
  Cos{1..4} (4 alike) : Trigonometry  Operator=cos
  Cos{5..8} (4 alike) : Trigonometry
  CruiseSlope_Deg : Constant  Value=0
  Divide : Product  Commented=on  Inputs=/*
  East : Constant  Value=90
  "East " : Constant  Value=90
  East 1 : Constant  Value=90
  East1 : Constant  Value=90
  Gain : Gain  Gain=-1
  Goto1 : Goto  Commented=on  GotoTag=ShortFinalFlag  TagVisibility=global
  Goto2 : Goto  Commented=on  GotoTag=FinalFlag  TagVisibility=global
  Minus{,1..7} (8 alike) : Sum  Inputs=+-
  Multiply : Product  Commented=on
  Multiply{1..8,10} (9 alike) : Product
  Multiply9 : Product  Commented=on
  NOT : Logic  Commented=on  Operator=NOT  IconShape=distinctive  AllPortsSameDT=off  OutDataTypeStr=boolean
  North : Constant  Value=0
  "North " : Constant  Value=0
  North 1 : Constant  Value=0
  North1 : Constant  Value=0
  Saturation : Saturate  UpperLimit=AltMax  LowerLimit=TerrainHeight*0.3048
  Saturation1 : Saturate  UpperLimit=100  LowerLimit=-100
  Saturation2 : Saturate  Commented=on  UpperLimit=AltMax  LowerLimit=ShortFinalHeight
  Sin : Trigonometry  Commented=on
  Sin1 : Trigonometry  Commented=on  Operator=atan
  Sin2 : Trigonometry  Commented=on
  Sin3 : Trigonometry
  Subtract : Sum  Commented=on  Inputs=+-
  Subtract1 : Sum  Commented=on  Inputs=-+
  Subtract2 : Sum  Commented=on  Inputs=-+
  Sum{1..8} (8 alike) : Sum  Inputs=|++
  Sum10 : Sum  Commented=on  Inputs=+-|
  Sum9 : Sum  Commented=on  Inputs=|+-
  Switch1 : Switch  Criteria=u2 > Threshold
  Switch2 : Switch  Commented=on  Criteria=u2 > Threshold
  Switch3 : Switch  Criteria=u2 > Threshold
  Switch4 : Switch  Criteria=u2 > Threshold
  deg2rad{1..8} (8 alike) : Gain  Gain=pi/180
  ft2m1 : Gain  Commented=on  Gain=0.3048
  Sim.Xpos : Outport
  Sim.Vx : Outport  Port=2
  Sim.Ypos : Outport  Port=3
  Sim.Vy : Outport  Port=4
  Sim.Zpos : Outport  Port=5
  Sim.Vz : Outport  Port=6
  wires:
  Multiply4/1 -> Sum4/2  "EastVelocity2LonVelocity"
  VNorth_mps/1 -> Multiply3/2, Multiply1/2
  Cos2/1 -> Multiply2/1
  Constant14/1 -> Switch3/1
  Switch4/1 -> Sin3/1
  Constant9/1 -> ft2m1/1
  Minus/1 -> deg2rad2/1
  Constant6/1 -> Subtract/2
  Add/1 -> Sum10/2
  Sum9/1 -> Saturation2/1
  Cos3/1 -> Multiply6/1
  Sum4/1 -> Sim.Vx/1  "Sim.Vx"
  Sum1/1 -> Minus2/1, Minus3/1  "Direction of Lateral Track"
  deg2rad4/1 -> Cos4/1
  Sum6/1 -> Minus/1, Minus1/1  "Direction of Lateral Track"
  Constant12/1 -> Add/2
  Minus5/1 -> deg2rad5/1
  VEast_mps/1 -> Multiply4/2, Multiply2/2
  Sum10/1 -> Switch3/2, Compare To Constant2/1, Switch2/2, Multiply9/2
  Gain/1 -> Multiply10/1
  North/1 -> Minus/2
  Sum3/1 -> Minus6/1, Minus7/1  "Direction of Lon Track"
  Minus3/1 -> deg2rad3/1
  CruiseSlope_Deg/1 -> Switch4/3
  TrackHeading_Deg/1 -> Sum6/1, Sum3/1, Sum5/1, Sum1/1
  Multiply10/1 -> Switch1/1
  Multiply5/1 -> Sum8/1  "NorthPosn2LonPosn"
  Saturation2/1 -> Subtract2/2, Switch2/3
  Multiply7/1 -> Sum7/2  "EastPosn2LateralPosn"
  Multiply8/1 -> Sum8/2  "EastPosn2LonPosn"
  Minus2/1 -> deg2rad4/1
  Xposn_m/1 -> Multiply5/2, Multiply6/2
  Multiply6/1 -> Sum7/1  "NorthPosn2LateralPosn"
  Multiply/1 -> Sum9/2
  Multiply1/1 -> Sum2/1  "NorthVelocity2LateralVelocity"
  Sin2/1 -> Multiply9/1
  Constant1/1 -> Sum1/2
  NOT/1 -> Goto1/1
  Compare To Constant1/1 -> Switch4/2, Switch1/2, Goto2/1
  "North "/1 -> Minus2/2
  Multiply3/1 -> Sum4/1  "NorthVelocity2LonVelocity"
  Switch1/1 -> Saturation1/1
  Yposn_m/1 -> Multiply7/2, Multiply8/2
  Constant/1 -> Saturation/1
  ft2m1/1 -> Subtract1/2, Sum9/1
  Switch3/1 -> Switch4/1
  North 1/1 -> Minus6/2
  Subtract/1 -> Multiply/1
  Compare To Constant2/1 -> NOT/1
  deg2rad8/1 -> Cos8/1
  Subtract1/1 -> Divide/2
  Sin/1 -> Multiply/2
  deg2rad2/1 -> Cos3/1
  Sin3/1 -> Multiply10/2
  Constant10/1 -> Subtract1/1
  Sum5/1 -> Minus4/1, Minus5/1  "Direction of Lon Track"
  Constant13/1 -> Switch3/3
  Saturation/1 -> Sim.Zpos/1  "Sim.Zpos"
  Multiply2/1 -> Sum2/2  "EastVelocity2LateralVelocity"
  Constant5/1 -> Switch1/3
  East1/1 -> Minus5/2
  Minus4/1 -> deg2rad6/1
  Sum8/1 -> Sim.Xpos/1, Sum10/1, Compare To Constant1/1, Subtract/1  "Sim.Xpos"
  Sum2/1 -> Sim.Vy/1  "Sim.Vy"
  Switch2/1 -> ?
  East/1 -> Minus1/2
  Cos7/1 -> Multiply5/1
  Cos1/1 -> Multiply7/1
  Minus7/1 -> deg2rad7/1
  Constant7/1 -> Sin/1
  deg2rad3/1 -> Cos2/1
  North1/1 -> Minus4/2
  Cos6/1 -> Multiply4/1
  deg2rad1/1 -> Cos1/1
  Cos4/1 -> Multiply1/1
  "East "/1 -> Minus3/2
  Minus6/1 -> deg2rad8/1
  deg2rad7/1 -> Cos6/1
  deg2rad5/1 -> Cos5/1
  Constant2/1 -> Sum3/2
  Cos5/1 -> Multiply8/1
  Constant4/1 -> Sum6/2
  Cos8/1 -> Multiply3/1
  Constant3/1 -> Sum5/2
  East 1/1 -> Minus7/2
  Constant11/1 -> Sin1/1
  Sin1/1 -> Divide/1
  Multiply9/1 -> Subtract2/1
  Minus1/1 -> deg2rad1/1
  Subtract2/1 -> Switch2/1
  Constant8/1 -> Sin2/1
  deg2rad6/1 -> Cos7/1
  Divide/1 -> Add/1
  Saturation1/1 -> Sim.Vz/1  "Sim.Vz"
  VGround_mps/1 -> Gain/1
  Sum7/1 -> Sim.Ypos/1  "Sim.Ypos"
